simulink model "teststuff"  (R2023a)
settings: Solver=VariableStepAuto  StartTime=0.0  StopTime=10.0  RelTol=1e-3
settings Model: Creator=Franz  LastModifiedBy=Franz

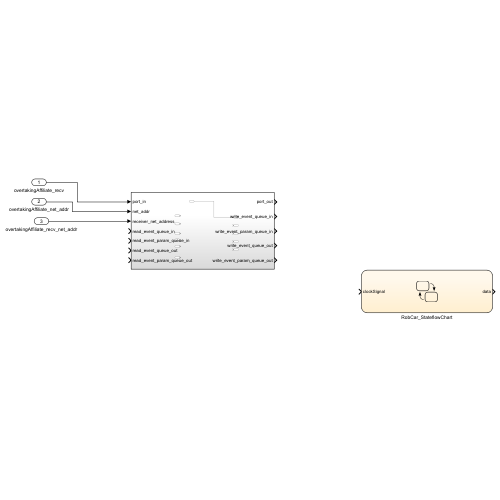
[thumbnail: Simulink's stored preview of the top-level diagram]
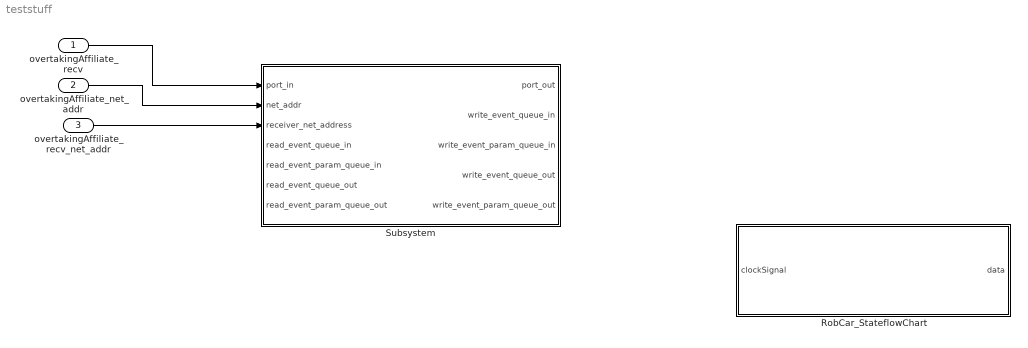
== system teststuff ==
  overtakingAffiliate_recv : Inport
  overtakingAffiliate_net_addr : Inport  Port=2
  overtakingAffiliate_recv_net_addr : Inport  Port=3
  RobCar_StateflowChart : Stateflow chart  TreatAsAtomicUnit=on
  Subsystem : Subsystem
  wires:
  overtakingAffiliate_recv_net_addr/1 -> Subsystem/3(receiver_net_address)
  overtakingAffiliate_recv/1 -> Subsystem/1(port_in)
  overtakingAffiliate_net_addr/1 -> Subsystem/2(net_addr)

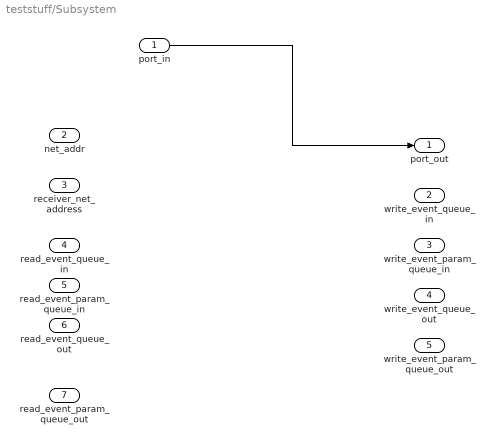
== system teststuff/Subsystem ==
  port_in : Inport
  net_addr : Inport  Port=2
  receiver_net_address : Inport  Port=3
  read_event_queue_in : Inport  Port=4
  read_event_param_queue_in : Inport  Port=5
  read_event_queue_out : Inport  Port=6
  read_event_param_queue_out : Inport  Port=7
  port_out : Outport
  write_event_queue_in : Outport  Port=2
  write_event_param_queue_in : Outport  Port=3
  write_event_queue_out : Outport  Port=4
  write_event_param_queue_out : Outport  Port=5
  wires:
  port_in/1 -> port_out/1

== stateflow chart teststuff/RobCar_StateflowChart ==
  data: data output; clockSignal input
